simulink model "TST_DuringActionTest"  (Simulink 7.4)
settings: Solver=FixedStepDiscrete  StartTime=0.0  StopTime=10.0  FixedStep=0.02  RelTol=1e-3
settings Model: Creator=kharthforeign  LastModifiedBy=kharthforeign  BufferReuse=off
settings DataIOCC: SaveOutput=off  SignalLogging=off  SaveTime=off
settings OptimizationCC: BlockReduction=off  ConditionallyExecuteInputs=off  OptimizeBlockIOStorage=off  BufferReuse=off  ExpressionFolding=off  LocalBlockOutputs=off  InitFltsAndDblsToZero=on
settings RTWCC: GenCodeOnly=on

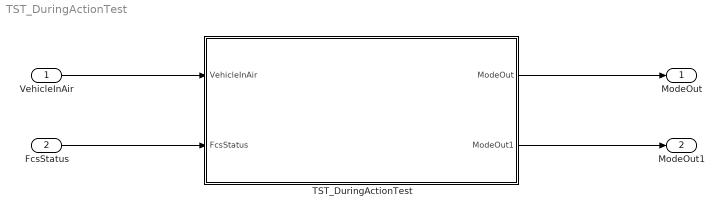
== system TST_DuringActionTest ==
  VehicleInAir : Inport  PortDimensions=1  DataType=boolean  OutDataType=fixdt(1, 16)  OutScaling=2^0  OutDataTypeStr=boolean
  FcsStatus : Inport  Port=2  UseBusObject=on  OutDataType=fixdt(1, 16)  OutScaling=2^0
      settings: BusObject=FCS_FlightControlSystem_Status
  TST_DuringActionTest : Subsystem  TreatAsAtomicUnit=on
  ModeOut : Outport  PortDimensions=1  DataType=int32  OutDataType=Enum: GBL_Definitions_EjectionCmd  OutDataTypeStr=int32
  ModeOut1 : Outport  Port=2  PortDimensions=1  DataType=int32  OutDataType=Enum: GBL_Definitions_EjectionCmd  OutDataTypeStr=int32
  wires:
  VehicleInAir/1 -> TST_DuringActionTest/1(VehicleInAir)
  FcsStatus/1 -> TST_DuringActionTest/2(FcsStatus)
  TST_DuringActionTest/1(ModeOut) -> ModeOut/1
  TST_DuringActionTest/2(ModeOut1) -> ModeOut1/1

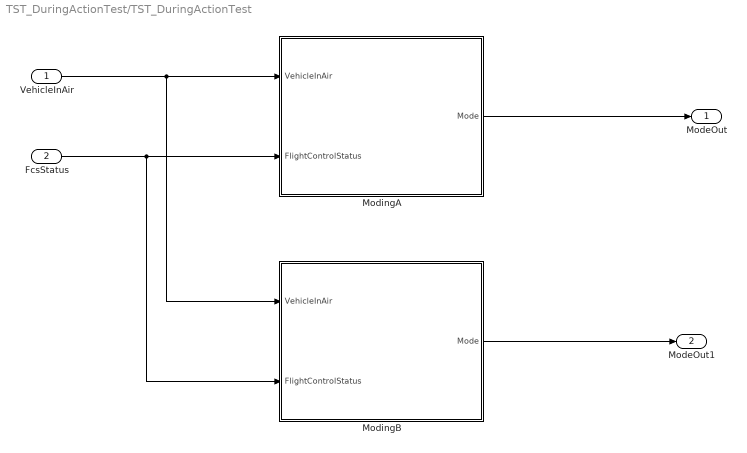
== system TST_DuringActionTest/TST_DuringActionTest ==
  VehicleInAir : Inport  PortDimensions=1  DataType=boolean  OutDataType=fixdt(1, 16)  OutScaling=2^0  OutDataTypeStr=boolean
  FcsStatus : Inport  Port=2  UseBusObject=on  OutDataType=fixdt(1, 16)  OutScaling=2^0
      settings: BusObject=FCS_FlightControlSystem_Status
  ModingA : Stateflow chart  TreatAsAtomicUnit=on
  ModingB : Stateflow chart  TreatAsAtomicUnit=on
  ModeOut : Outport  PortDimensions=1  DataType=int32  OutDataType=Enum: GBL_Definitions_EjectionCmd  OutDataTypeStr=int32
  ModeOut1 : Outport  Port=2  PortDimensions=1  DataType=int32  OutDataType=Enum: GBL_Definitions_EjectionCmd  OutDataTypeStr=int32
  wires:
  FcsStatus/1 -> ModingA/2(FlightControlStatus), ModingB/2(FlightControlStatus)
  VehicleInAir/1 -> ModingA/1(VehicleInAir), ModingB/1(VehicleInAir)
  ModingA/1(Mode) -> ModeOut/1
  ModingB/1(Mode) -> ModeOut1/1

== stateflow chart TST_DuringActionTest/ModingA ==
  state TopStateA
    during:
    Mode = int32(111);
    state Autoland
      entry:
      Mode = int32(3);
      during:
      Mode = int32(-3);
    state Off
      entry:
      Mode = int32(1);
    state Launch
      entry:
      Mode = int32(2);
    (default) -> Off
    Launch -> Autoland : [(FlightControlStatus.PressureAltitude_Ft > 1500.0) || VehicleInAir]
    Off -> Launch : [(FlightControlStatus.PressureAltitude_Ft < 500.0) && (~VehicleInAir)]
  state TopStateB
    during:
    Mode = int32(222);
  (default) -> TopStateA
  TopStateA -> TopStateB : [Mode >= int32(123)]
  data: VehicleInAir input boolean; Mode output int32; FlightControlStatus input FCS_FlightControlSystem_Status

== stateflow chart TST_DuringActionTest/ModingB ==
  state TopStateA
    during:
    Mode = int32(111);
    state Autoland
      entry:
      Mode = int32(3);
      during:
      Mode = int32(-3);
    state Off
      entry:
      Mode = int32(1);
    state Launch
      entry:
      Mode = int32(2);
      during:
      Mode = int32(-2);
    (default) -> Off
    Launch -> Autoland [order 1] : [FlightControlStatus.PressureAltitude_Ft > 1500.0]
    Off -> Launch : [(FlightControlStatus.PressureAltitude_Ft < 500.0) && (~VehicleInAir)]
  state TopStateB
    during:
    Mode = int32(222);
  (default) -> TopStateA
  TopStateA -> TopStateB : [Mode >= int32(123)]
  Launch -> TopStateB [order 2] : [VehicleInAir]
  TopStateB -> TopStateA
  data: VehicleInAir input boolean; Mode output int32; FlightControlStatus input FCS_FlightControlSystem_Status
